simulink model "EcoSIM3_P2_C2_WIP"  (R2014b)
settings: Solver=ode1  SolverMode=SingleTasking  StartTime=0.0  StopTime=4  FixedStep=0.01  RelTol=1e-3
PostLoadFcn:
  | %, if any(exist('dsrtsu_mdlpostloadfcn', 'file') == [2, 3, 6]), try dsrtsu_mdlpostloadfcn('Execute', bdroot); catch fprintf('Error in PostLoadFcn (dsrtsu_mdlpostloadfcn) for model "%s":\n %s\n', bdroot, lasterr); end, end,
InitFcn:
  | tic
  | %Startup_EcoSIM
undefined symbols (not defined in the file or in its folder): canChannel, Controls, DriveCycles, Driver, EM_EFF_MAP, EM_PwrLoss_MAP, EngPwr, EngSpd, EngTrq, Glbl, Overwritten_Mode, Plants, Power, sigbuilder_block, Torque, Trialmap, Veh_Dynamics
libraries: simulink x135, canmsglib x113, fl_lib x104, canlib x89, nesl_utility x56, sdl_lib x29, dspsigops x6, dspswit3 x5, dspstat3 x2, commnoisgen2 x1, dspfdesign x1
(part 13 of 21)

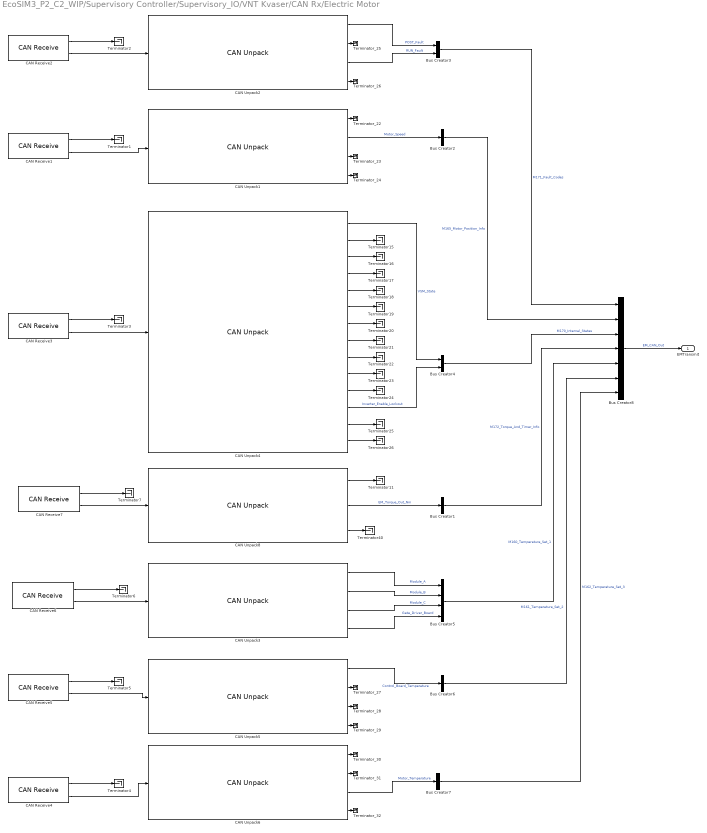
== system EcoSIM3_P2_C2_WIP/Supervisory Controller/Supervisory_IO/VNT Kvaser/CAN Rx/Electric Motor ==
  Bus Creator{1..2,6..7} (4 alike) : BusCreator  Inputs=1
  Bus Creator3 : BusCreator  Inputs=2
  Bus Creator4 : BusCreator  Inputs=2
  Bus Creator5 : BusCreator
  Bus Creator8 : BusCreator  Inputs=7
  CAN Receive1 : canlib/CAN Receive  BlockHandle=7472.0023  DeviceMenu=Kvaser Virtual 1 (Channel 2)  Device=Kvaser Virtual 1 (Channel 2)  ObjConstructor=canChannel('Kvaser', 'Virtual 1', 2)  EnableStandardIDsFilter=off  StandardIDs=165  EnableExtendedIDsFilter=off  ExtendedIDs=0  SampleTime=0.01  MsgsPerTimestep=1  StdIDsCombo=Allow only  ExtIDsCombo=Block all  InternalFilterUpdateStatus=on
  CAN Receive2 : canlib/CAN Receive  BlockHandle=7473.0023  DeviceMenu=Kvaser Virtual 1 (Channel 2)  Device=Kvaser Virtual 1 (Channel 2)  ObjConstructor=canChannel('Kvaser', 'Virtual 1', 2)  EnableStandardIDsFilter=off  StandardIDs=171  EnableExtendedIDsFilter=off  ExtendedIDs=0  SampleTime=0.01  MsgsPerTimestep=1  StdIDsCombo=Allow only  ExtIDsCombo=Block all  InternalFilterUpdateStatus=on
  CAN Receive3 : canlib/CAN Receive  BlockHandle=7474.0023  DeviceMenu=Kvaser Virtual 1 (Channel 2)  Device=Kvaser Virtual 1 (Channel 2)  ObjConstructor=canChannel('Kvaser', 'Virtual 1', 2)  EnableStandardIDsFilter=off  StandardIDs=170  EnableExtendedIDsFilter=off  ExtendedIDs=0  SampleTime=0.01  MsgsPerTimestep=1  StdIDsCombo=Allow only  ExtIDsCombo=Block all  InternalFilterUpdateStatus=on
  CAN Receive4 : canlib/CAN Receive  BlockHandle=7475.0023  DeviceMenu=Kvaser Virtual 1 (Channel 2)  Device=Kvaser Virtual 1 (Channel 2)  ObjConstructor=canChannel('Kvaser', 'Virtual 1', 2)  EnableStandardIDsFilter=off  StandardIDs=162  EnableExtendedIDsFilter=off  ExtendedIDs=0  SampleTime=0.01  MsgsPerTimestep=1  StdIDsCombo=Allow only  ExtIDsCombo=Block all  InternalFilterUpdateStatus=on
  CAN Receive5 : canlib/CAN Receive  BlockHandle=7476.0023  DeviceMenu=Kvaser Virtual 1 (Channel 2)  Device=Kvaser Virtual 1 (Channel 2)  ObjConstructor=canChannel('Kvaser', 'Virtual 1', 2)  EnableStandardIDsFilter=off  StandardIDs=161  EnableExtendedIDsFilter=off  ExtendedIDs=0  SampleTime=0.01  MsgsPerTimestep=1  StdIDsCombo=Allow only  ExtIDsCombo=Block all  InternalFilterUpdateStatus=on
  CAN Receive6 : canlib/CAN Receive  BlockHandle=7477.0023  DeviceMenu=Kvaser Virtual 1 (Channel 2)  Device=Kvaser Virtual 1 (Channel 2)  ObjConstructor=canChannel('Kvaser', 'Virtual 1', 2)  EnableStandardIDsFilter=off  StandardIDs=160  EnableExtendedIDsFilter=off  ExtendedIDs=0  SampleTime=0.01  MsgsPerTimestep=1  StdIDsCombo=Allow only  ExtIDsCombo=Block all  InternalFilterUpdateStatus=on
  CAN Receive7 : canlib/CAN Receive  BlockHandle=7478.0023  DeviceMenu=Kvaser Virtual 1 (Channel 2)  Device=Kvaser Virtual 1 (Channel 2)  ObjConstructor=canChannel('Kvaser', 'Virtual 1', 2)  EnableStandardIDsFilter=off  StandardIDs=172  EnableExtendedIDsFilter=off  ExtendedIDs=0  SampleTime=0.01  MsgsPerTimestep=1  StdIDsCombo=Allow only  ExtIDsCombo=Block all  InternalFilterUpdateStatus=on
  CAN Unpack1 : canmsglib/CAN Unpack  CANdbFile=C:\Users\EcoCAR_HIL\Documents\Khanna\EcoSIM3_P1_0_PHEV_TCU\Final_DBC\20150828 RMS PM CAN DB.dbc  MsgList=M165_Motor_Position_Info  MsgName=M165_Motor_Position_Info  MsgIDType=Standard (11-bit identifier)  MsgIdentifier=165  MsgLength=8  SignalInfo=D1_Motor_Angle_Electrical$0$16$1$2$1$0$1.000000e-01$0$0$6.553500e+03$#D2_Motor_Speed$16$16$1$1$1$0$1$0$-32768$32767$#D3_Electrical_Output_Frequency$32$16$1$1$1$0$1.000000e-01$0$-3.276800e+03$3.276700e+03$#D4_Delta_Resolver_Filtered$48$16$1$1$1$0$1.000000e-01$0$-3.276800e+03$3.276700e+03$#  NSignals=4  IDPort=off  TimestampPort=off  ErrorPort=off  RemotePort=off  LengthPort=off  StatusPort=off  StartBits=str2num('[int32(0);int32(16);int32(32);int32(48)]')  SignalSizes=str2num('[int32(16);int32(16);int32(16);int32(16)]')  ByteOrders=str2num('[int32(1);int32(1);int32(1);int32(1)]')  DataTypes=str2num('[int32(2);int32(1);int32(1);int32(1)]')  MultiplexTypes=str2num('[int32(1);int32(1);int32(1);int32(1)]')  MultiplexValues=str2num('[double(0);double(0);double(0);double(0)]')  Factors=str2num('[double(1.000000e-01);double(1);double(1.000000e-01);double(1.000000e-01)]')  Offsets=str2num('[double(0);double(0);double(0);double(0)]')  Minimums=str2num('[double(0);double(-32768);double(-3.276800e+03);double(-3.276800e+03)]')  Maximums=str2num('[double(6.553500e+03);double(32767);double(3.276700e+03);double(3.276700e+03)]')
      settings: DataFormat=CANdb specified signals
  CAN Unpack2 : canmsglib/CAN Unpack  CANdbFile=C:\Users\EcoCAR_HIL\Documents\Khanna\EcoSIM3_P1_0_PHEV_TCU\Final_DBC\20150828 RMS PM CAN DB.dbc  MsgList=M171_Fault_Codes  MsgName=M171_Fault_Codes  MsgIDType=Standard (11-bit identifier)  MsgIdentifier=171  MsgLength=8  SignalInfo=D1_Post_Fault_Lo$0$16$1$2$1$0$1$0$0$65535$#D2_Post_Fault_Hi$16$16$1$2$1$0$1$0$0$65535$#D3_Run_Fault_Lo$32$16$1$2$1$0$1$0$0$65535$#D4_Run_Fault_Hi$48$16$1$2$1$0$1$0$0$65535$#  NSignals=4  IDPort=off  TimestampPort=off  ErrorPort=off  RemotePort=off  LengthPort=off  StatusPort=off  StartBits=str2num('[int32(0);int32(16);int32(32);int32(48)]')  SignalSizes=str2num('[int32(16);int32(16);int32(16);int32(16)]')  ByteOrders=str2num('[int32(1);int32(1);int32(1);int32(1)]')  DataTypes=str2num('[int32(2);int32(2);int32(2);int32(2)]')  MultiplexTypes=str2num('[int32(1);int32(1);int32(1);int32(1)]')  MultiplexValues=str2num('[double(0);double(0);double(0);double(0)]')  Factors=str2num('[double(1);double(1);double(1);double(1)]')  Offsets=str2num('[double(0);double(0);double(0);double(0)]')  Minimums=str2num('[double(0);double(0);double(0);double(0)]')  Maximums=str2num('[double(65535);double(65535);double(65535);double(65535)]')
      settings: DataFormat=CANdb specified signals
  CAN Unpack3 : canmsglib/CAN Unpack  CANdbFile=C:\Users\EcoCAR_HIL\Documents\Khanna\EcoSIM3_P1_0_PHEV_TCU\Final_DBC\20150828 RMS PM CAN DB.dbc  MsgList=M160_Temperature_Set_1  MsgName=M160_Temperature_Set_1  MsgIDType=Standard (11-bit identifier)  MsgIdentifier=160  MsgLength=8  SignalInfo=D1_Module_A$0$16$1$1$1$0$1.000000e-01$0$-3.276800e+03$3.276700e+03$#D2_Module_B$16$16$1$1$1$0$1.000000e-01$0$-3.276800e+03$3.276700e+03$#D3_Module_C$32$16$1$1$1$0$1.000000e-01$0$-3.276800e+03$3.276700e+03$#D4_Gate_Driver_Board$48$16$1$1$1$0$1.000000e-01$0$-3.276800e+03$3.276700e+03$#  NSignals=4  IDPort=off  TimestampPort=off  ErrorPort=off  RemotePort=off  LengthPort=off  StatusPort=off  StartBits=str2num('[int32(0);int32(16);int32(32);int32(48)]')  SignalSizes=str2num('[int32(16);int32(16);int32(16);int32(16)]')  ByteOrders=str2num('[int32(1);int32(1);int32(1);int32(1)]')  DataTypes=str2num('[int32(1);int32(1);int32(1);int32(1)]')  MultiplexTypes=str2num('[int32(1);int32(1);int32(1);int32(1)]')  MultiplexValues=str2num('[double(0);double(0);double(0);double(0)]')  Factors=str2num('[double(1.000000e-01);double(1.000000e-01);double(1.000000e-01);double(1.000000e-01)]')  Offsets=str2num('[double(0);double(0);double(0);double(0)]')  Minimums=str2num('[double(-3.276800e+03);double(-3.276800e+03);double(-3.276800e+03);double(-3.276800e+03)]')  Maximums=str2num('[double(3.276700e+03);double(3.276700e+03);double(3.276700e+03);double(3.276700e+03)]')
      settings: DataFormat=CANdb specified signals
  CAN Unpack4 : canmsglib/CAN Unpack  CANdbFile=C:\Users\EcoCAR_HIL\Documents\Khanna\EcoSIM3_P1_0_PHEV_TCU\Final_DBC\20150828 RMS PM CAN DB.dbc  MsgList=M170_Internal_States  MsgName=M170_Internal_States  MsgIDType=Standard (11-bit identifier)  MsgIdentifier=170  MsgLength=8  SignalInfo=D1_VSM_State$0$16$1$2$1$0$1$0$0$15$#D2_Inverter_State$16$8$1$2$1$0$1$0$0$255$#D3_Relay_1_Status$24$1$1$2$1$0$1$0$0$1$#D3_Relay_2_Status$25$1$1$2$1$0$1$0$0$1$#D3_Relay_3_Status$26$1$1$2$1$0$1$0$0$1$#D3_Relay_4_Status$27$1$1$2$1$0$1$0$0$1$#D3_Relay_5_Status$28$1$1$2$1$0$1$0$-Inf$Inf$#D3_Relay_6_Status$29$1$1$2$1$0$1$0$-Inf$Inf$#D4_Inverter_Discharge_State$37$3$1$2$1$0$1$0$0$7$#D4_Inverter_Run_Mode$32$1$1$2$1$0$1$0$0$1$#D5_Inverter_Command_Mode$40$1$1$2$1$0$1$0$0$1$#D6_Inverter_Enable_Lockout$55$1$1$2$1$0$1$0$0$1$#D6_Inverter_Enable_State$48$1$1$2$1$0$1$0$0$1$#D7_Direction_Command$56$8$1$2$1$0$1$0$0$1$#  NSignals=14  IDPort=off  TimestampPort=off  ErrorPort=off  RemotePort=off  LengthPort=off  StatusPort=off  StartBits=str2num('[int32(0);int32(16);int32(24);int32(25);int32(26);int32(27);int32(28);int32(29);int32(37);int32(32);int32(40);int32(55);int32(48);int32(56)]')  SignalSizes=str2num('[int32(16);int32(8);int32(1);int32(1);int32(1);int32(1);int32(1);int32(1);int32(3);int32(1);int32(1);int32(1);int32(1);int32(8)]')  ByteOrders=str2num('[int32(1);int32(1);int32(1);int32(1);int32(1);int32(1);int32(1);int32(1);int32(1);int32(1);int32(1);int32(1);int32(1);int32(1)]')  DataTypes=str2num('[int32(2);int32(2);int32(2);int32(2);int32(2);int32(2);int32(2);int32(2);int32(2);int32(2);int32(2);int32(2);int32(2);int32(2)]')  MultiplexTypes=str2num('[int32(1);int32(1);int32(1);int32(1);int32(1);int32(1);int32(1);int32(1);int32(1);int32(1);int32(1);int32(1);int32(1);int32(1)]')  MultiplexValues=str2num('[double(0);double(0);double(0);double(0);double(0);double(0);double(0);double(0);double(0);double(0);double(0);double(0);double(0);double(0)]')  Factors=str2num('[double(1);double(1);double(1);double(1);double(1);double(1);double(1);double(1);double(1);double(1);double(1);double(1);double(1);double(1)]')  Offsets=str2num('[double(0);double(0);double(0);double(0);double(0);double(0);double(0);double(0);double(0);double(0);double(0);double(0);double(0);double(0)]')  Minimums=str2num('[double(0);double(0);double(0);double(0);double(0);double(0);double(-Inf);double(-Inf);double(0);double(0);double(0);double(0);double(0);double(0)]')  Maximums=str2num('[double(15);double(255);double(1);double(1);double(1);double(1);double(Inf);double(Inf);double(7);double(1);double(1);double(1);double(1);double(1)]')
      settings: DataFormat=CANdb specified signals
  CAN Unpack5 : canmsglib/CAN Unpack  CANdbFile=C:\Users\EcoCAR_HIL\Documents\Khanna\EcoSIM3_P1_0_PHEV_TCU\Final_DBC\20150828 RMS PM CAN DB.dbc  MsgList=M161_Temperature_Set_2  MsgName=M161_Temperature_Set_2  MsgIDType=Standard (11-bit identifier)  MsgIdentifier=161  MsgLength=8  SignalInfo=D1_Control_Board_Temperature$0$16$1$1$1$0$1.000000e-01$0$-3.276800e+03$3.276700e+03$#D2_RTD1_Temperature$16$16$1$1$1$0$1.000000e-01$0$-3.276800e+03$3.276700e+03$#D3_RTD2_Temperature$32$16$1$1$1$0$1.000000e-01$0$-3.276800e+03$3.276700e+03$#D4_RTD3_Temperature$48$16$1$1$1$0$1.000000e-01$0$-3.276800e+03$3.276700e+03$#  NSignals=4  IDPort=off  TimestampPort=off  ErrorPort=off  RemotePort=off  LengthPort=off  StatusPort=off  StartBits=str2num('[int32(0);int32(16);int32(32);int32(48)]')  SignalSizes=str2num('[int32(16);int32(16);int32(16);int32(16)]')  ByteOrders=str2num('[int32(1);int32(1);int32(1);int32(1)]')  DataTypes=str2num('[int32(1);int32(1);int32(1);int32(1)]')  MultiplexTypes=str2num('[int32(1);int32(1);int32(1);int32(1)]')  MultiplexValues=str2num('[double(0);double(0);double(0);double(0)]')  Factors=str2num('[double(1.000000e-01);double(1.000000e-01);double(1.000000e-01);double(1.000000e-01)]')  Offsets=str2num('[double(0);double(0);double(0);double(0)]')  Minimums=str2num('[double(-3.276800e+03);double(-3.276800e+03);double(-3.276800e+03);double(-3.276800e+03)]')  Maximums=str2num('[double(3.276700e+03);double(3.276700e+03);double(3.276700e+03);double(3.276700e+03)]')
      settings: DataFormat=CANdb specified signals
  CAN Unpack6 : canmsglib/CAN Unpack  CANdbFile=C:\Users\EcoCAR_HIL\Documents\Khanna\EcoSIM3_P1_0_PHEV_TCU\Final_DBC\20150828 RMS PM CAN DB.dbc  MsgList=M162_Temperature_Set_3  MsgName=M162_Temperature_Set_3  MsgIDType=Standard (11-bit identifier)  MsgIdentifier=162  MsgLength=8  SignalInfo=D1_RTD4_Temperature$0$16$1$1$1$0$1.000000e-01$0$-3.276800e+03$3.276700e+03$#D2_RTD5_Temperature$16$16$1$1$1$0$1.000000e-01$0$-3.276800e+03$3.276700e+03$#D3_Motor_Temperature$32$16$1$1$1$0$1.000000e-01$0$-3.276800e+03$3.276700e+03$#D4_Torque_Shudder$48$16$1$1$1$0$1.000000e-01$0$-3.276800e+03$3.276700e+03$#  NSignals=4  IDPort=off  TimestampPort=off  ErrorPort=off  RemotePort=off  LengthPort=off  StatusPort=off  StartBits=str2num('[int32(0);int32(16);int32(32);int32(48)]')  SignalSizes=str2num('[int32(16);int32(16);int32(16);int32(16)]')  ByteOrders=str2num('[int32(1);int32(1);int32(1);int32(1)]')  DataTypes=str2num('[int32(1);int32(1);int32(1);int32(1)]')  MultiplexTypes=str2num('[int32(1);int32(1);int32(1);int32(1)]')  MultiplexValues=str2num('[double(0);double(0);double(0);double(0)]')  Factors=str2num('[double(1.000000e-01);double(1.000000e-01);double(1.000000e-01);double(1.000000e-01)]')  Offsets=str2num('[double(0);double(0);double(0);double(0)]')  Minimums=str2num('[double(-3.276800e+03);double(-3.276800e+03);double(-3.276800e+03);double(-3.276800e+03)]')  Maximums=str2num('[double(3.276700e+03);double(3.276700e+03);double(3.276700e+03);double(3.276700e+03)]')
      settings: DataFormat=CANdb specified signals
  CAN Unpack8 : canmsglib/CAN Unpack  CANdbFile=C:\Users\EcoCAR_HIL\Documents\Khanna\EcoSIM3_P1_0_PHEV_TCU\Final_DBC\20150828 RMS PM CAN DB.dbc  MsgList=M172_Torque_And_Timer_Info  MsgName=M172_Torque_And_Timer_Info  MsgIDType=Standard (11-bit identifier)  MsgIdentifier=172  MsgLength=8  SignalInfo=D1_Commanded_Torque$0$16$1$1$1$0$1.000000e-01$0$-3.276800e+03$3.276700e+03$#D2_Torque_Feedback$16$16$1$1$1$0$1.000000e-01$0$-3.276800e+03$3.276700e+03$#D3_Power_On_Timer$32$32$1$2$1$0$3.000000e-03$0$0$4294970000$#  NSignals=3  IDPort=off  TimestampPort=off  ErrorPort=off  RemotePort=off  LengthPort=off  StatusPort=off  StartBits=str2num('[int32(0);int32(16);int32(32)]')  SignalSizes=str2num('[int32(16);int32(16);int32(32)]')  ByteOrders=str2num('[int32(1);int32(1);int32(1)]')  DataTypes=str2num('[int32(1);int32(1);int32(2)]')  MultiplexTypes=str2num('[int32(1);int32(1);int32(1)]')  MultiplexValues=str2num('[double(0);double(0);double(0)]')  Factors=str2num('[double(1.000000e-01);double(1.000000e-01);double(3.000000e-03)]')  Offsets=str2num('[double(0);double(0);double(0)]')  Minimums=str2num('[double(-3.276800e+03);double(-3.276800e+03);double(0)]')  Maximums=str2num('[double(3.276700e+03);double(3.276700e+03);double(4294970000)]')
      settings: DataFormat=CANdb specified signals
  Terminator{1..7,11,15..26,40} (21 alike) : Terminator
  Terminator_{22..32} (11 alike) : Terminator
  EMTransmit : Outport
  wires:
  Bus Creator4/1 -> Bus Creator8/3  "M170_Internal_States"
  CAN Unpack4/1 -> Bus Creator4/1  "VSM_State"
  CAN Unpack4/2 -> Terminator15/1
  CAN Unpack4/3 -> Terminator16/1
  CAN Unpack4/4 -> Terminator17/1
  CAN Unpack4/5 -> Terminator18/1
  CAN Unpack4/6 -> Terminator19/1
  CAN Unpack4/7 -> Terminator20/1
  CAN Unpack4/8 -> Terminator21/1
  CAN Unpack4/9 -> Terminator22/1
  CAN Unpack4/10 -> Terminator23/1
  CAN Unpack4/11 -> Terminator24/1
  CAN Unpack4/13 -> Terminator25/1
  CAN Unpack4/14 -> Terminator26/1
  CAN Unpack8/1 -> Terminator11/1
  CAN Unpack8/3 -> Terminator40/1
  CAN Unpack4/12 -> Bus Creator4/2  "Inverter_Enable_Lockout"
  CAN Unpack8/2 -> Bus Creator1/1  "EM_Torque_Out_Nm"
  CAN Receive1/1 -> Terminator1/1
  CAN Unpack1/2 -> Bus Creator2/1  "Motor_Speed"
  CAN Unpack2/1 -> Bus Creator3/1  "POST_Fault"
  CAN Unpack2/3 -> Bus Creator3/2  "RUN_Fault"
  CAN Unpack3/1 -> Bus Creator5/1  "Module_A"
  CAN Unpack3/2 -> Bus Creator5/2  "Module_B"
  CAN Unpack3/3 -> Bus Creator5/3  "Module_C"
  CAN Unpack3/4 -> Bus Creator5/4  "Gate_Driver_Board"
  CAN Unpack5/1 -> Bus Creator6/1  "Control_Board_Temperature"
  CAN Unpack6/3 -> Bus Creator7/1  "Motor_Temperature"
  Bus Creator3/1 -> Bus Creator8/1  "M171_Fault_Codes"
  Bus Creator2/1 -> Bus Creator8/2  "M165_Motor_Position_Info"
  Bus Creator1/1 -> Bus Creator8/4  "M172_Torque_And_Timer_Info"
  Bus Creator5/1 -> Bus Creator8/5  "M160_Temperature_Set_1"
  Bus Creator6/1 -> Bus Creator8/6  "M161_Temperature_Set_2"
  Bus Creator7/1 -> Bus Creator8/7  "M162_Temperature_Set_3"
  Bus Creator8/1 -> EMTransmit/1  "EM_CAN_Out"
  CAN Unpack1/1 -> Terminator_22/1
  CAN Unpack1/3 -> Terminator_23/1
  CAN Unpack1/4 -> Terminator_24/1
  CAN Unpack2/2 -> Terminator_25/1
  CAN Unpack2/4 -> Terminator_26/1
  CAN Unpack5/2 -> Terminator_27/1
  CAN Unpack5/3 -> Terminator_28/1
  CAN Unpack5/4 -> Terminator_29/1
  CAN Unpack6/1 -> Terminator_30/1
  CAN Unpack6/2 -> Terminator_31/1
  CAN Unpack6/4 -> Terminator_32/1
  CAN Receive2/1 -> Terminator2/1
  CAN Receive3/1 -> Terminator3/1
  CAN Receive4/1 -> Terminator4/1
  CAN Receive5/1 -> Terminator5/1
  CAN Receive6/1 -> Terminator6/1
  CAN Receive7/1 -> Terminator7/1
  CAN Receive2/2 -> CAN Unpack2/1
  CAN Receive1/2 -> CAN Unpack1/1
  CAN Receive7/2 -> CAN Unpack8/1
  CAN Receive6/2 -> CAN Unpack3/1
  CAN Receive5/2 -> CAN Unpack5/1
  CAN Receive3/2 -> CAN Unpack4/1
  CAN Receive4/2 -> CAN Unpack6/1

== system EcoSIM3_P2_C2_WIP/Supervisory Controller/Supervisory_IO/VNT Kvaser/CAN Rx/Engine ==
  Bus Creator : BusCreator  Inputs=1
  Bus Creator4 : BusCreator  Inputs=1
  CAN Receive1 : canlib/CAN Receive  BlockHandle=7581.0027  DeviceMenu=Kvaser Virtual 1 (Channel 1)  Device=Kvaser Virtual 1 (Channel 1)  ObjConstructor=canChannel('Kvaser', 'Virtual 1', 1)  EnableStandardIDsFilter=off  StandardIDs=104  EnableExtendedIDsFilter=off  ExtendedIDs=0  SampleTime=0.01  MsgsPerTimestep=1  StdIDsCombo=Allow only  ExtIDsCombo=Block all  InternalFilterUpdateStatus=on
  CAN Unpack1 : canmsglib/CAN Unpack  CANdbFile=C:\Users\EcoCAR_HIL\Documents\Khanna\EcoSIM3_P1_0_PHEV_TCU\Final_DBC\Engine_Transmission_BAS.dbc  MsgList=ECO_Engine_MSG104  MsgName=ECO_Engine_MSG104  MsgIDType=Standard (11-bit identifier)  MsgIdentifier=104  MsgLength=2  SignalInfo=ICE_Torque_Cmd_Nm$9$15$2$2$1$0$1.000000e-02$0$0$3.276700e+02$#  NSignals=1  IDPort=off  TimestampPort=off  ErrorPort=off  RemotePort=off  LengthPort=off  StatusPort=off  StartBits=str2num('[int32(9)]')  SignalSizes=str2num('[int32(15)]')  ByteOrders=str2num('[int32(2)]')  DataTypes=str2num('[int32(2)]')  MultiplexTypes=str2num('[int32(1)]')  MultiplexValues=str2num('[double(0)]')  Factors=str2num('[double(1.000000e-02)]')  Offsets=str2num('[double(0)]')  Minimums=str2num('[double(0)]')  Maximums=str2num('[double(3.276700e+02)]')
      settings: DataFormat=CANdb specified signals
  Terminator1 : Terminator
  ICETransmit : Outport
  wires:
  CAN Receive1/2 -> CAN Unpack1/1
  CAN Receive1/1 -> Terminator1/1
  CAN Unpack1/1 -> Bus Creator/1  "ICE_Torque_Cmd_Nm"
  Bus Creator/1 -> Bus Creator4/1  "ICE_Torque"
  Bus Creator4/1 -> ICETransmit/1  "ICE_CAN_Out"

== system EcoSIM3_P2_C2_WIP/Supervisory Controller/Supervisory_IO/VNT Kvaser/CAN Rx/GCM ==
  Bus Creator7 : BusCreator  Inputs=1
  CAN Receive9 : canlib/CAN Receive  BlockHandle=7592.0027  DeviceMenu=Kvaser Virtual 1 (Channel 1)  Device=Kvaser Virtual 1 (Channel 1)  ObjConstructor=canChannel('Kvaser', 'Virtual 1', 1)  EnableStandardIDsFilter=off  StandardIDs=96  EnableExtendedIDsFilter=off  ExtendedIDs=0  SampleTime=0.01  MsgsPerTimestep=1  StdIDsCombo=Allow only  ExtIDsCombo=Block all  InternalFilterUpdateStatus=on
  CAN Unpack9 : canmsglib/CAN Unpack  CANdbFile=C:\Users\EcoCAR_HIL\Documents\Khanna\EcoSIM3_P1_0_PHEV_TCU\Final_DBC\EcoCAR3_Controls_Development.dbc  MsgList=GCM_Transmit_MSG096  MsgName=GCM_Transmit_MSG096  MsgIDType=Standard (11-bit identifier)  MsgIdentifier=96  MsgLength=1  SignalInfo=charge_mode_request$7$1$2$2$1$0$1$0$0$1$#  NSignals=1  IDPort=off  TimestampPort=off  ErrorPort=off  RemotePort=off  LengthPort=off  StatusPort=off  StartBits=str2num('[int32(7)]')  SignalSizes=str2num('[int32(1)]')  ByteOrders=str2num('[int32(2)]')  DataTypes=str2num('[int32(2)]')  MultiplexTypes=str2num('[int32(1)]')  MultiplexValues=str2num('[double(0)]')  Factors=str2num('[double(1)]')  Offsets=str2num('[double(0)]')  Minimums=str2num('[double(0)]')  Maximums=str2num('[double(1)]')
      settings: DataFormat=CANdb specified signals
  Terminator10 : Terminator
  FromGCM : Outport
  wires:
  CAN Receive9/2 -> CAN Unpack9/1
  CAN Receive9/1 -> Terminator10/1
  CAN Unpack9/1 -> Bus Creator7/1  "charge_mode_request"
  Bus Creator7/1 -> FromGCM/1  "GCM_CAN_Out"

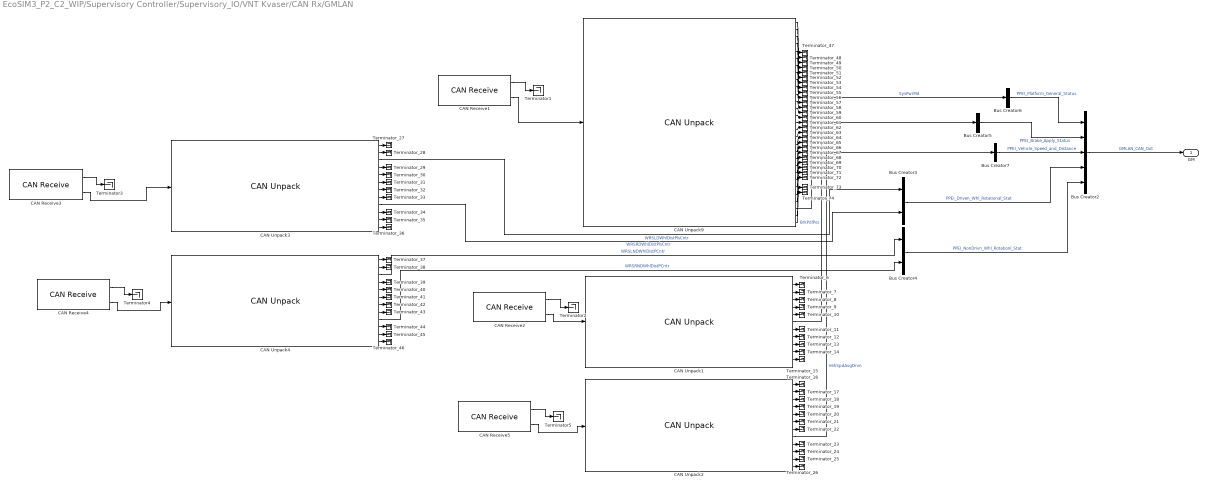
== system EcoSIM3_P2_C2_WIP/Supervisory Controller/Supervisory_IO/VNT Kvaser/CAN Rx/GMLAN ==
  Bus Creator2 : BusCreator  Inputs=5
  Bus Creator3 : BusCreator  Inputs=2
  Bus Creator4 : BusCreator  Inputs=2
  Bus Creator5 : BusCreator  Inputs=1
  Bus Creator6 : BusCreator  Inputs=1
  Bus Creator7 : BusCreator  Inputs=1
  CAN Receive1 : canlib/CAN Receive  BlockHandle=7607.0027  DeviceMenu=Kvaser Virtual 1 (Channel 1)  Device=Kvaser Virtual 1 (Channel 1)  ObjConstructor=canChannel('Kvaser', 'Virtual 1', 1)  EnableStandardIDsFilter=off  StandardIDs=497  EnableExtendedIDsFilter=off  ExtendedIDs=0  SampleTime=0.01  MsgsPerTimestep=1  StdIDsCombo=Allow only  ExtIDsCombo=Block all  InternalFilterUpdateStatus=on
  CAN Receive2 : canlib/CAN Receive  BlockHandle=7608.0023  DeviceMenu=Kvaser Virtual 1 (Channel 1)  Device=Kvaser Virtual 1 (Channel 1)  ObjConstructor=canChannel('Kvaser', 'Virtual 1', 1)  EnableStandardIDsFilter=off  StandardIDs=241  EnableExtendedIDsFilter=off  ExtendedIDs=0  SampleTime=0.01  MsgsPerTimestep=1  StdIDsCombo=Allow only  ExtIDsCombo=Block all  InternalFilterUpdateStatus=on
  CAN Receive3 : canlib/CAN Receive  BlockHandle=7609.0023  DeviceMenu=Kvaser Virtual 1 (Channel 1)  Device=Kvaser Virtual 1 (Channel 1)  ObjConstructor=canChannel('Kvaser', 'Virtual 1', 1)  EnableStandardIDsFilter=off  StandardIDs=193  EnableExtendedIDsFilter=off  ExtendedIDs=0  SampleTime=0.01  MsgsPerTimestep=1  StdIDsCombo=Allow only  ExtIDsCombo=Block all  InternalFilterUpdateStatus=on
  CAN Receive4 : canlib/CAN Receive  BlockHandle=7610.0023  DeviceMenu=Kvaser Virtual 1 (Channel 1)  Device=Kvaser Virtual 1 (Channel 1)  ObjConstructor=canChannel('Kvaser', 'Virtual 1', 1)  EnableStandardIDsFilter=off  StandardIDs=197  EnableExtendedIDsFilter=off  ExtendedIDs=0  SampleTime=0.01  MsgsPerTimestep=1  StdIDsCombo=Allow only  ExtIDsCombo=Block all  InternalFilterUpdateStatus=on
  CAN Receive5 : canlib/CAN Receive  BlockHandle=7611.0023  DeviceMenu=Kvaser Virtual 1 (Channel 1)  Device=Kvaser Virtual 1 (Channel 1)  ObjConstructor=canChannel('Kvaser', 'Virtual 1', 1)  EnableStandardIDsFilter=off  StandardIDs=1001  EnableExtendedIDsFilter=off  ExtendedIDs=0  SampleTime=0.01  MsgsPerTimestep=1  StdIDsCombo=Allow only  ExtIDsCombo=Block all  InternalFilterUpdateStatus=on
  CAN Unpack1 : canmsglib/CAN Unpack  CANdbFile=C:\Users\EcoCAR_HIL\Documents\Khanna\EcoSIM3_P1_0_PHEV_TCU\Final_DBC\GlobalAHS_anon GM CONFIDENTIAL.dbc  MsgList=PPEI_Brake_Apply_Status  MsgName=PPEI_Brake_Apply_Status  MsgIDType=Standard (11-bit identifier)  MsgIdentifier=241  MsgLength=6  SignalInfo=BrkAppSnsrHmPosLrnd$30$1$2$2$1$0$1$0$0$1$#BrkPdlChkData$40$17$2$2$1$0$1$0$0$131071$#BrkPdlInTrvPrt$2$2$2$2$1$0$1$0$0$3$#BrkPdlModTrvl$6$1$2$2$1$0$1$0$0$1$#BrkPdlModTrvlV$7$1$2$2$1$0$1$0$0$1$#BrkPdlPos$8$8$2$2$1$0$3.921570e-01$0$0$1.000000e+02$#BrkPdlPosGrad$16$8$2$1$1$0$40$0$-5120$5080$#BrkPedPosAlvRolngCnt$4$2$2$2$1$0$1$0$0$3$#BrkPedTrvlAchvd$1$1$2$2$1$0$1$0$0$1$#BrkPedTrvlAchvdV$0$1$2$2$1$0$1$0$0$1$#NotEventStat$28$2$2$2$1$0$1$0$0$3$#  NSignals=11  IDPort=off  TimestampPort=off  ErrorPort=off  RemotePort=off  LengthPort=off  StatusPort=off  StartBits=str2num('[int32(30);int32(40);int32(2);int32(6);int32(7);int32(8);int32(16);int32(4);int32(1);int32(0);int32(28)]')  SignalSizes=str2num('[int32(1);int32(17);int32(2);int32(1);int32(1);int32(8);int32(8);int32(2);int32(1);int32(1);int32(2)]')  ByteOrders=str2num('[int32(2);int32(2);int32(2);int32(2);int32(2);int32(2);int32(2);int32(2);int32(2);int32(2);int32(2)]')  DataTypes=str2num('[int32(2);int32(2);int32(2);int32(2);int32(2);int32(2);int32(1);int32(2);int32(2);int32(2);int32(2)]')  MultiplexTypes=str2num('[int32(1);int32(1);int32(1);int32(1);int32(1);int32(1);int32(1);int32(1);int32(1);int32(1);int32(1)]')  MultiplexValues=str2num('[double(0);double(0);double(0);double(0);double(0);double(0);double(0);double(0);double(0);double(0);double(0)]')  Factors=str2num('[double(1);double(1);double(1);double(1);double(1);double(3.921570e-01);double(40);double(1);double(1);double(1);double(1)]')  Offsets=str2num('[double(0);double(0);double(0);double(0);double(0);double(0);double(0);double(0);double(0);double(0);double(0)]')  Minimums=str2num('[double(0);double(0);double(0);double(0);double(0);double(0);double(-5120);double(0);double(0);double(0);double(0)]')  Maximums=str2num('[double(1);double(131071);double(3);double(1);double(1);double(1.000000e+02);double(5080);double(3);double(1);double(1);double(3)]')
      settings: DataFormat=CANdb specified signals
  CAN Unpack2 : canmsglib/CAN Unpack  CANdbFile=C:\Users\EcoCAR_HIL\Documents\Khanna\EcoSIM3_P1_0_PHEV_TCU\Final_DBC\GlobalAHS_anon GM CONFIDENTIAL.dbc  MsgList=PPEI_Vehicle_Speed_and_Distance  MsgName=PPEI_Vehicle_Speed_and_Distance  MsgIDType=Standard (11-bit identifier)  MsgIdentifier=1001  MsgLength=8  SignalInfo=DistRollCntAvgDrvn$24$13$2$2$1$0$1.250000e-01$0$0$1.023875e+03$#DistRollCntAvgDrvnSrc$55$1$2$2$1$0$1$0$0$1$#DistRollCntAvgDrvnV$22$1$2$2$1$0$1$0$0$1$#DstRolCntAvNDrRstOc$53$1$2$2$1$0$1$0$0$1$#DstRolCntAvgDrnRstOc$21$1$2$2$1$0$1$0$0$1$#DstRolCntAvgNonDrvn$56$13$2$2$1$0$1.250000e-01$0$0$1.023875e+03$#DstRolCntAvgNonDrvnV$54$1$2$2$1$0$1$0$0$1$#VehSpdAvgDrvn$8$15$2$2$1$0$1.562500e-02$0$0$5.119844e+02$#VehSpdAvgDrvnSrc$23$1$2$2$1$0$1$0$0$1$#VehSpdAvgDrvnV$7$1$2$2$1$0$1$0$0$1$#VehSpdAvgNDrvn$40$15$2$2$1$0$1.562500e-02$0$0$5.119844e+02$#VehSpdAvgNDrvnV$39$1$2$2$1$0$1$0$0$1$#  NSignals=12  IDPort=off  TimestampPort=off  ErrorPort=off  RemotePort=off  LengthPort=off  StatusPort=off  StartBits=str2num('[int32(24);int32(55);int32(22);int32(53);int32(21);int32(56);int32(54);int32(8);int32(23);int32(7);int32(40);int32(39)]')  SignalSizes=str2num('[int32(13);int32(1);int32(1);int32(1);int32(1);int32(13);int32(1);int32(15);int32(1);int32(1);int32(15);int32(1)]')  ByteOrders=str2num('[int32(2);int32(2);int32(2);int32(2);int32(2);int32(2);int32(2);int32(2);int32(2);int32(2);int32(2);int32(2)]')  DataTypes=str2num('[int32(2);int32(2);int32(2);int32(2);int32(2);int32(2);int32(2);int32(2);int32(2);int32(2);int32(2);int32(2)]')  MultiplexTypes=str2num('[int32(1);int32(1);int32(1);int32(1);int32(1);int32(1);int32(1);int32(1);int32(1);int32(1);int32(1);int32(1)]')  MultiplexValues=str2num('[double(0);double(0);double(0);double(0);double(0);double(0);double(0);double(0);double(0);double(0);double(0);double(0)]')  Factors=str2num('[double(1.250000e-01);double(1);double(1);double(1);double(1);double(1.250000e-01);double(1);double(1.562500e-02);double(1);double(1);double(1.562500e-02);double(1)]')  Offsets=str2num('[double(0);double(0);double(0);double(0);double(0);double(0);double(0);double(0);double(0);double(0);double(0);double(0)]')  Minimums=str2num('[double(0);double(0);double(0);double(0);double(0);double(0);double(0);double(0);double(0);double(0);double(0);double(0)]')  Maximums=str2num('[double(1.023875e+03);double(1);double(1);double(1);double(1);double(1.023875e+03);double(1);double(5.119844e+02);double(1);double(1);double(5.119844e+02);double(1)]')
      settings: DataFormat=CANdb specified signals
  CAN Unpack3 : canmsglib/CAN Unpack  CANdbFile=C:\Users\EcoCAR_HIL\Documents\Khanna\EcoSIM3_P1_0_PHEV_TCU\Final_DBC\GlobalAHS_anon GM CONFIDENTIAL.dbc  MsgList=PPEI_Driven_Whl_Rotational_Stat  MsgName=PPEI_Driven_Whl_Rotational_Stat  MsgIDType=Standard (11-bit identifier)  MsgIdentifier=193  MsgLength=8  SignalInfo=WRSLDSeqNum$4$2$2$2$1$0$1$0$0$3$#WRSLDWhlDisTpRC$6$2$2$2$1$0$1$0$0$3$#WRSLDWhlDistPlsCntr$8$10$2$2$1$0$1$0$0$1023$#WRSLDWhlDistTmstm$24$16$2$2$1$0$1$0$0$65535$#WRSLDWhlDistVal$2$1$2$2$1$0$1$0$0$1$#WRSLDWhlRotStatRst$3$1$2$2$1$0$1$0$0$1$#WRSRDSeqNum$36$2$2$2$1$0$1$0$0$3$#WRSRDWhlDisTpRC$38$2$2$2$1$0$1$0$0$3$#WRSRDWhlDistPlsCntr$40$10$2$2$1$0$1$0$0$1023$#WRSRDWhlDistTmstm$56$16$2$2$1$0$1$0$0$65535$#WRSRDWhlDistVal$34$1$2$2$1$0$1$0$0$1$#WRSRDWhlRotStatRst$35$1$2$2$1$0$1$0$0$1$#  NSignals=12  IDPort=off  TimestampPort=off  ErrorPort=off  RemotePort=off  LengthPort=off  StatusPort=off  StartBits=str2num('[int32(4);int32(6);int32(8);int32(24);int32(2);int32(3);int32(36);int32(38);int32(40);int32(56);int32(34);int32(35)]')  SignalSizes=str2num('[int32(2);int32(2);int32(10);int32(16);int32(1);int32(1);int32(2);int32(2);int32(10);int32(16);int32(1);int32(1)]')  ByteOrders=str2num('[int32(2);int32(2);int32(2);int32(2);int32(2);int32(2);int32(2);int32(2);int32(2);int32(2);int32(2);int32(2)]')  DataTypes=str2num('[int32(2);int32(2);int32(2);int32(2);int32(2);int32(2);int32(2);int32(2);int32(2);int32(2);int32(2);int32(2)]')  MultiplexTypes=str2num('[int32(1);int32(1);int32(1);int32(1);int32(1);int32(1);int32(1);int32(1);int32(1);int32(1);int32(1);int32(1)]')  MultiplexValues=str2num('[double(0);double(0);double(0);double(0);double(0);double(0);double(0);double(0);double(0);double(0);double(0);double(0)]')  Factors=str2num('[double(1);double(1);double(1);double(1);double(1);double(1);double(1);double(1);double(1);double(1);double(1);double(1)]')  Offsets=str2num('[double(0);double(0);double(0);double(0);double(0);double(0);double(0);double(0);double(0);double(0);double(0);double(0)]')  Minimums=str2num('[double(0);double(0);double(0);double(0);double(0);double(0);double(0);double(0);double(0);double(0);double(0);double(0)]')  Maximums=str2num('[double(3);double(3);double(1023);double(65535);double(1);double(1);double(3);double(3);double(1023);double(65535);double(1);double(1)]')
      settings: DataFormat=CANdb specified signals
  CAN Unpack4 : canmsglib/CAN Unpack  CANdbFile=C:\Users\EcoCAR_HIL\Documents\Khanna\EcoSIM3_P1_0_PHEV_TCU\Final_DBC\GlobalAHS_anon GM CONFIDENTIAL.dbc  MsgList=PPEI_NonDrivn_Whl_Rotationl_Stat  MsgName=PPEI_NonDrivn_Whl_Rotationl_Stat  MsgIDType=Standard (11-bit identifier)  MsgIdentifier=197  MsgLength=8  SignalInfo=WRSLNDSeqNum$4$2$2$2$1$0$1$0$0$3$#WRSLNDWhlDisTpRC$6$2$2$2$1$0$1$0$0$3$#WRSLNDWhlDistPCntr$8$10$2$2$1$0$1$0$0$1023$#WRSLNDWhlDistTstm$24$16$2$2$1$0$1$0$0$65535$#WRSLNDWhlDistVal$2$1$2$2$1$0$1$0$0$1$#WRSLNDWhlRotStRst$3$1$2$2$1$0$1$0$0$1$#WRSRNDSeqNum$36$2$2$2$1$0$1$0$0$3$#WRSRNDWhlDisTpRC$38$2$2$2$1$0$1$0$0$3$#WRSRNDWhlDistPCntr$40$10$2$2$1$0$1$0$0$1023$#WRSRNDWhlDistTstm$56$16$2$2$1$0$1$0$0$65535$#WRSRNDWhlDistVal$34$1$2$2$1$0$1$0$0$1$#WRSRNDWhlRotStRst$35$1$2$2$1$0$1$0$0$1$#  NSignals=12  IDPort=off  TimestampPort=off  ErrorPort=off  RemotePort=off  LengthPort=off  StatusPort=off  StartBits=str2num('[int32(4);int32(6);int32(8);int32(24);int32(2);int32(3);int32(36);int32(38);int32(40);int32(56);int32(34);int32(35)]')  SignalSizes=str2num('[int32(2);int32(2);int32(10);int32(16);int32(1);int32(1);int32(2);int32(2);int32(10);int32(16);int32(1);int32(1)]')  ByteOrders=str2num('[int32(2);int32(2);int32(2);int32(2);int32(2);int32(2);int32(2);int32(2);int32(2);int32(2);int32(2);int32(2)]')  DataTypes=str2num('[int32(2);int32(2);int32(2);int32(2);int32(2);int32(2);int32(2);int32(2);int32(2);int32(2);int32(2);int32(2)]')  MultiplexTypes=str2num('[int32(1);int32(1);int32(1);int32(1);int32(1);int32(1);int32(1);int32(1);int32(1);int32(1);int32(1);int32(1)]')  MultiplexValues=str2num('[double(0);double(0);double(0);double(0);double(0);double(0);double(0);double(0);double(0);double(0);double(0);double(0)]')  Factors=str2num('[double(1);double(1);double(1);double(1);double(1);double(1);double(1);double(1);double(1);double(1);double(1);double(1)]')  Offsets=str2num('[double(0);double(0);double(0);double(0);double(0);double(0);double(0);double(0);double(0);double(0);double(0);double(0)]')  Minimums=str2num('[double(0);double(0);double(0);double(0);double(0);double(0);double(0);double(0);double(0);double(0);double(0);double(0)]')  Maximums=str2num('[double(3);double(3);double(1023);double(65535);double(1);double(1);double(3);double(3);double(1023);double(65535);double(1);double(1)]')
      settings: DataFormat=CANdb specified signals
  CAN Unpack9 : canmsglib/CAN Unpack  CANdbFile=C:\Users\EcoCAR_HIL\Documents\Khanna\EcoSIM3_P1_0_PHEV_TCU\Final_DBC\GlobalAHS_anon GM CONFIDENTIAL.dbc  MsgList=PPEI_Platform_General_Status  MsgName=PPEI_Platform_General_Status  MsgIDType=Standard (11-bit identifier)  MsgIdentifier=497  MsgLength=8  SignalInfo=ACCmpsrFldOn$63$1$2$2$1$0$1$0$0$1$#ACCompModReq$11$2$2$2$1$0$1$0$0$3$#ACCompNormLd$48$8$2$2$1$0$1.000000e-01$0$0$2.550000e+01$#ACCompNormLdV$10$1$2$2$1$0$1$0$0$1$#ACCompSysVDA$9$1$2$2$1$0$1$0$0$1$#ACCompSysVDM$60$1$2$2$1$0$1$0$0$1$#AirbgVDA$57$1$2$2$1$0$1$0$0$1$#BkupPwrModeMstrVDA$7$1$2$2$1$0$1$0$0$1$#BkupPwrModeMstrVDM$61$1$2$2$1$0$1$0$0$1$#DispMeasSys$59$1$2$2$1$0$1$0$0$1$#ElvtdIdlCstStReq$32$2$2$2$1$0$1$0$0$3$#EngOilLfRstRq$37$1$2$2$1$0$1$0$0$1$#FuelFltLfRstRqd$56$1$2$2$1$0$1$0$0$1$#ImmblzrPreRelPswdStat$8$1$2$2$1$0$1$0$0$1$#ImmblzrPreRelPswrd$24$16$2$2$1$0$1$0$0$65535$#PMMAccTrmSt$2$1$2$2$1$0$1$0$0$1$#PMMRunCrkTrmSt$3$1$2$2$1$0$1$0$0$1$#PTORSMstrEngShtReq$13$1$2$2$1$0$1$0$0$1$#PTORmStMsEngStRq$14$1$2$2$1$0$1$0$0$1$#PrkBrkSwAtv$36$1$2$2$1$0$1$0$0$1$#PrkBrkVDA$35$1$2$2$1$0$1$0$0$1$#PrkBrkVDM$62$1$2$2$1$0$1$0$0$1$#RmVehStrRq$15$1$2$2$1$0$1$0$0$1$#SIRDpl$58$1$2$2$1$0$1$0$0$1$#SysBkUpPwrMd$4$2$2$2$1$0$1$0$0$3$#SysBkupPwrMdEn$6$1$2$2$1$0$1$0$0$1$#SysPwrMd$0$2$2$2$1$0$1$0$0$3$#ThrtlPrgrsnReq$38$2$2$2$1$0$1$0$0$3$#TrStLgMdAtv$34$1$2$2$1$0$1$0$0$1$#  NSignals=29  IDPort=off  TimestampPort=off  ErrorPort=off  RemotePort=off  LengthPort=off  StatusPort=off  StartBits=str2num('[int32(63);int32(11);int32(48);int32(10);int32(9);int32(60);int32(57);int32(7);int32(61);int32(59);int32(32);int32(37);int32(56);int32(8);int32(24);int32(2);int32(3);int32(13);int32(14);int32(36);int32(35);int32(62);int32(15);int32(58);int32(4);int32(6);int32(0);int32(38);int32(34)]')  SignalSizes=str2num('[int32(1);int32(2);int32(8);int32(1);int32(1);int32(1);int32(1);int32(1);int32(1);int32(1);int32(2);int32(1);int32(1);int32(1);int32(16);int32(1);int32(1);int32(1);int32(1);int32(1);int32(1);int32(1);int32(1);int32(1);int32(2);int32(1);int32(2);int32(2);int32(1)]')  ByteOrders=str2num('[int32(2);int32(2);int32(2);int32(2);int32(2);int32(2);int32(2);int32(2);int32(2);int32(2);int32(2);int32(2);int32(2);int32(2);int32(2);int32(2);int32(2);int32(2);int32(2);int32(2);int32(2);int32(2);int32(2);int32(2);int32(2);int32(2);int32(2);int32(2);int32(2)]')  DataTypes=str2num('[int32(2);int32(2);int32(2);int32(2);int32(2);int32(2);int32(2);int32(2);int32(2);int32(2);int32(2);int32(2);int32(2);int32(2);int32(2);int32(2);int32(2);int32(2);int32(2);int32(2);int32(2);int32(2);int32(2);int32(2);int32(2);int32(2);int32(2);int32(2);int32(2)]')  MultiplexTypes=str2num('[int32(1);int32(1);int32(1);int32(1);int32(1);int32(1);int32(1);int32(1);int32(1);int32(1);int32(1);int32(1);int32(1);int32(1);int32(1);int32(1);int32(1);int32(1);int32(1);int32(1);int32(1);int32(1);int32(1);int32(1);int32(1);int32(1);int32(1);int32(1);int32(1)]')  MultiplexValues=str2num('[double(0);double(0);double(0);double(0);double(0);double(0);double(0);double(0);double(0);double(0);double(0);double(0);double(0);double(0);double(0);double(0);double(0);double(0);double(0);double(0);double(0);double(0);double(0);double(0);double(0);double(0);double(0);double(0);double(0)]')  Factors=str2num('[double(1);double(1);double(1.000000e-01);double(1);double(1);double(1);double(1);double(1);double(1);double(1);double(1);double(1);double(1);double(1);double(1);double(1);double(1);double(1);double(1);double(1);double(1);double(1);double(1);double(1);double(1);double(1);double(1);double(1);double(1)]')  Offsets=str2num('[double(0);double(0);double(0);double(0);double(0);double(0);double(0);double(0);double(0);double(0);double(0);double(0);double(0);double(0);double(0);double(0);double(0);double(0);double(0);double(0);double(0);double(0);double(0);double(0);double(0);double(0);double(0);double(0);double(0)]')  Minimums=str2num('[double(0);double(0);double(0);double(0);double(0);double(0);double(0);double(0);double(0);double(0);double(0);double(0);double(0);double(0);double(0);double(0);double(0);double(0);double(0);double(0);double(0);double(0);double(0);double(0);double(0);double(0);double(0);double(0);double(0)]')  Maximums=str2num('[double(1);double(3);double(2.550000e+01);double(1);double(1);double(1);double(1);double(1);double(1);double(1);double(3);double(1);double(1);double(1);double(65535);double(1);double(1);double(1);double(1);double(1);double(1);double(1);double(1);double(1);double(3);double(1);double(3);double(3);double(1)]')
      settings: DataFormat=CANdb specified signals
  Terminator{1..5} (5 alike) : Terminator
  Terminator_{6..74} (69 alike) : Terminator
  GM : Outport
  wires:
  CAN Unpack4/3 -> Bus Creator4/1  "WRSLNDWhlDistPCntr"
  CAN Unpack3/3 -> Bus Creator3/1  "WRSLDWhlDistPlsCntr"
  Bus Creator4/1 -> Bus Creator2/5  "PPEI_NonDrivn_Whl_Rotationl_Stat"
  Bus Creator3/1 -> Bus Creator2/4  "PPEI_Driven_Whl_Rotational_Stat"
  CAN Unpack4/9 -> Bus Creator4/2  "WRSRNDWhlDistPCntr"
  CAN Unpack3/9 -> Bus Creator3/2  "WRSRDWhlDistPlsCntr"
  Bus Creator2/1 -> GM/1  "GMLAN_CAN_Out"
  Bus Creator5/1 -> Bus Creator2/2  "PPEI_Brake_Apply_Status"
  Bus Creator6/1 -> Bus Creator2/1  "PPEI_Platform_General_Status"
  CAN Unpack2/8 -> Bus Creator7/1  "VehSpdAvgDrvn"
  Bus Creator7/1 -> Bus Creator2/3  "PPEI_Vehicle_Speed_and_Distance"
  CAN Unpack1/6 -> Bus Creator5/1  "BrkPdlPos"
  CAN Unpack9/27 -> Bus Creator6/1  "SysPwrMd"
  CAN Receive3/1 -> Terminator3/1
  CAN Unpack1/1 -> Terminator_6/1
  CAN Unpack1/2 -> Terminator_7/1
  CAN Unpack1/3 -> Terminator_8/1
  CAN Unpack1/4 -> Terminator_9/1
  CAN Unpack1/5 -> Terminator_10/1
  CAN Unpack1/7 -> Terminator_11/1
  CAN Unpack1/8 -> Terminator_12/1
  CAN Unpack1/9 -> Terminator_13/1
  CAN Unpack1/10 -> Terminator_14/1
  CAN Unpack1/11 -> Terminator_15/1
  CAN Unpack2/1 -> Terminator_16/1
  CAN Unpack2/2 -> Terminator_17/1
  CAN Unpack2/3 -> Terminator_18/1
  CAN Unpack2/4 -> Terminator_19/1
  CAN Unpack2/5 -> Terminator_20/1
  CAN Unpack2/6 -> Terminator_21/1
  CAN Unpack2/7 -> Terminator_22/1
  CAN Unpack2/9 -> Terminator_23/1
  CAN Unpack2/10 -> Terminator_24/1
  CAN Unpack2/11 -> Terminator_25/1
  CAN Unpack2/12 -> Terminator_26/1
  CAN Unpack3/1 -> Terminator_27/1
  CAN Unpack3/2 -> Terminator_28/1
  CAN Unpack3/4 -> Terminator_29/1
  CAN Unpack3/5 -> Terminator_30/1
  CAN Unpack3/6 -> Terminator_31/1
  CAN Unpack3/7 -> Terminator_32/1
  CAN Unpack3/8 -> Terminator_33/1
  CAN Unpack3/10 -> Terminator_34/1
  CAN Unpack3/11 -> Terminator_35/1
  CAN Unpack3/12 -> Terminator_36/1
  CAN Unpack4/1 -> Terminator_37/1
  CAN Unpack4/2 -> Terminator_38/1
  CAN Unpack4/4 -> Terminator_39/1
  CAN Unpack4/5 -> Terminator_40/1
  CAN Unpack4/6 -> Terminator_41/1
  CAN Unpack4/7 -> Terminator_42/1
  CAN Unpack4/8 -> Terminator_43/1
  CAN Unpack4/10 -> Terminator_44/1
  CAN Unpack4/11 -> Terminator_45/1
  CAN Unpack4/12 -> Terminator_46/1
  CAN Unpack9/1 -> Terminator_47/1
  CAN Unpack9/2 -> Terminator_48/1
  CAN Unpack9/3 -> Terminator_49/1
  CAN Unpack9/4 -> Terminator_50/1
  CAN Unpack9/5 -> Terminator_51/1
  CAN Unpack9/6 -> Terminator_52/1
  CAN Unpack9/7 -> Terminator_53/1
  CAN Unpack9/8 -> Terminator_54/1
  CAN Unpack9/9 -> Terminator_55/1
  CAN Unpack9/10 -> Terminator_56/1
  CAN Unpack9/11 -> Terminator_57/1
  CAN Unpack9/12 -> Terminator_58/1
  CAN Unpack9/13 -> Terminator_59/1
  CAN Unpack9/14 -> Terminator_60/1
  CAN Unpack9/15 -> Terminator_61/1
  CAN Unpack9/16 -> Terminator_62/1
  CAN Unpack9/17 -> Terminator_63/1
  CAN Unpack9/18 -> Terminator_64/1
  CAN Unpack9/19 -> Terminator_65/1
  CAN Unpack9/20 -> Terminator_66/1
  CAN Unpack9/21 -> Terminator_67/1
  CAN Unpack9/22 -> Terminator_68/1
  CAN Unpack9/23 -> Terminator_69/1
  CAN Unpack9/24 -> Terminator_70/1
  CAN Unpack9/25 -> Terminator_71/1
  CAN Unpack9/26 -> Terminator_72/1
  CAN Unpack9/28 -> Terminator_73/1
  CAN Unpack9/29 -> Terminator_74/1
  CAN Receive1/1 -> Terminator1/1
  CAN Receive2/1 -> Terminator2/1
  CAN Receive4/1 -> Terminator4/1
  CAN Receive5/1 -> Terminator5/1
  CAN Receive3/2 -> CAN Unpack3/1
  CAN Receive1/2 -> CAN Unpack9/1
  CAN Receive4/2 -> CAN Unpack4/1
  CAN Receive2/2 -> CAN Unpack1/1
  CAN Receive5/2 -> CAN Unpack2/1

== system EcoSIM3_P2_C2_WIP/Supervisory Controller/Supervisory_IO/VNT Kvaser/CAN Tx/ESS ==
  ESS : Inport
  Bus Selector2 : BusSelector  OutputSignals=ESS_Signals_A123.hsc_bcm_enable,ESS_Signals_A123.hsc_bcm_epo,ESS_Signals_A123.hsc_bcm_leakage_ena,ESS_Signals_A123.hsc_bcm_mainc_close
  CAN Pack4 : canmsglib/CAN Pack  CANdbFile=C:\Users\EcoCAR_HIL\Documents\Khanna\EcoSIM3_P1_0_PHEV_TCU\Final_DBC\BCM_VehBus_Std.dbc  MsgList=BCM_Request  MsgName=BCM_Request  MsgIDType=Standard (11-bit identifier)  MsgIdentifier=1024  MsgLength=4  SignalInfo=hsc_bcm_enable$0$1$2$2$1$0$1$0$0$1$#hsc_bcm_epo$1$1$2$2$1$0$1$0$0$1$#hsc_bcm_leakage_ena$3$1$2$2$1$0$1$0$0$1$#hsc_bcm_mainc_close$2$1$2$2$1$0$1$0$0$1$#  NSignals=4  StartBits=str2num('[int32(0);int32(1);int32(3);int32(2)]')  SignalSizes=str2num('[int32(1);int32(1);int32(1);int32(1)]')  ByteOrders=str2num('[int32(2);int32(2);int32(2);int32(2)]')  DataTypes=str2num('[int32(2);int32(2);int32(2);int32(2)]')  MultiplexTypes=str2num('[int32(1);int32(1);int32(1);int32(1)]')  MultiplexValues=str2num('[double(0);double(0);double(0);double(0)]')  Factors=str2num('[double(1);double(1);double(1);double(1)]')  Offsets=str2num('[double(0);double(0);double(0);double(0)]')  Minimums=str2num('[double(0);double(0);double(0);double(0)]')  Maximums=str2num('[double(1);double(1);double(1);double(1)]')  Remote=off
      settings: DataFormat=CANdb specified signals
  CAN Transmit4 : canlib/CAN Transmit  BlockHandle=7799.0023  DeviceMenu=Kvaser Virtual 1 (Channel 1)  Device=Kvaser Virtual 1 (Channel 1)  ObjConstructor=canChannel('Kvaser', 'Virtual 1', 1)  EnablePeriodicTransmit=off  MessagePeriod=1.000
  Rate Transition{,1..3} (4 alike) : RateTransition
  wires:
  ESS/1 -> Bus Selector2/1
  Bus Selector2/2 -> Rate Transition1/1  "<hsc_bcm_epo>"
  Bus Selector2/3 -> Rate Transition2/1  "<hsc_bcm_leakage_ena>"
  CAN Pack4/1 -> CAN Transmit4/1
  Bus Selector2/4 -> Rate Transition3/1  "<hsc_bcm_mainc_close>"
  Bus Selector2/1 -> Rate Transition/1  "<hsc_bcm_enable>"
  Rate Transition/1 -> CAN Pack4/1
  Rate Transition1/1 -> CAN Pack4/2
  Rate Transition2/1 -> CAN Pack4/3
  Rate Transition3/1 -> CAN Pack4/4

== system EcoSIM3_P2_C2_WIP/Supervisory Controller/Supervisory_IO/VNT Kvaser/CAN Tx/Eelctric Motor ==
  EMTransmit : Inport
  Bus Selector : BusSelector  OutputSignals=Rotation_Direction,Inverter_Enable,Torque_Command
  Bus Selector1 : BusSelector  OutputSignals=EM_Messages_Rhinehart
  CAN Pack : canmsglib/CAN Pack  CANdbFile=C:\Users\EcoCAR_HIL\Documents\Khanna\EcoSIM3_P1_0_PHEV_TCU\Final_DBC\20150828 RMS PM CAN DB.dbc  MsgList=M192_Command_Message  MsgName=M192_Command_Message  MsgIDType=Standard (11-bit identifier)  MsgIdentifier=192  MsgLength=8  SignalInfo=Direction_Command$42$1$1$2$1$0$1$0$0$1$#Inverter_Discharge$41$1$1$2$1$0$1$0$0$1$#Inverter_Enable$40$1$1$2$1$0$1$0$0$1$#Speed_Command$16$16$1$1$1$0$1$0$-32768$32767$#Torque_Command$0$16$1$1$1$0$1.000000e-01$0$-3.276800e+03$3.276700e+03$#Torque_Limit_Command$48$16$1$1$1$0$1$0$-3.276800e+03$3.276700e+03$#  NSignals=6  StartBits=str2num('[int32(42);int32(41);int32(40);int32(16);int32(0);int32(48)]')  SignalSizes=str2num('[int32(1);int32(1);int32(1);int32(16);int32(16);int32(16)]')  ByteOrders=str2num('[int32(1);int32(1);int32(1);int32(1);int32(1);int32(1)]')  DataTypes=str2num('[int32(2);int32(2);int32(2);int32(1);int32(1);int32(1)]')  MultiplexTypes=str2num('[int32(1);int32(1);int32(1);int32(1);int32(1);int32(1)]')  MultiplexValues=str2num('[double(0);double(0);double(0);double(0);double(0);double(0)]')  Factors=str2num('[double(1);double(1);double(1);double(1);double(1.000000e-01);double(1)]')  Offsets=str2num('[double(0);double(0);double(0);double(0);double(0);double(0)]')  Minimums=str2num('[double(0);double(0);double(0);double(-32768);double(-3.276800e+03);double(-3.276800e+03)]')  Maximums=str2num('[double(1);double(1);double(1);double(32767);double(3.276700e+03);double(3.276700e+03)]')  Remote=off
      settings: DataFormat=CANdb specified signals
  CAN Transmit : canlib/CAN Transmit  BlockHandle=7819.0023  DeviceMenu=Kvaser Virtual 1 (Channel 2)  Device=Kvaser Virtual 1 (Channel 2)  ObjConstructor=canChannel('Kvaser', 'Virtual 1', 2)  EnablePeriodicTransmit=off  MessagePeriod=1.000
  Ground : Ground
  Ground2 : Ground
  Ground3 : Ground
  Rate Transition : RateTransition
  Rate Transition1 : RateTransition
  Rate Transition2 : RateTransition
  wires:
  EMTransmit/1 -> Bus Selector1/1
  Bus Selector/2 -> Rate Transition1/1  "<Inverter_Enable>"
  Ground3/1 -> CAN Pack/6
  Ground2/1 -> CAN Pack/4
  Ground/1 -> CAN Pack/2
  Bus Selector/3 -> Rate Transition2/1  "<Torque_Command>"
  Bus Selector/1 -> Rate Transition/1  "<Rotation_Direction>"
  CAN Pack/1 -> CAN Transmit/1
  Bus Selector1/1 -> Bus Selector/1  "<EM_Messages_Rhinehart>"
  Rate Transition/1 -> CAN Pack/1
  Rate Transition1/1 -> CAN Pack/3
  Rate Transition2/1 -> CAN Pack/5
